simulink model "Ex2s"  (R2025a)
settings: Solver=VariableStepAuto  StartTime=0.0  StopTime=4  RelTol=1e-3

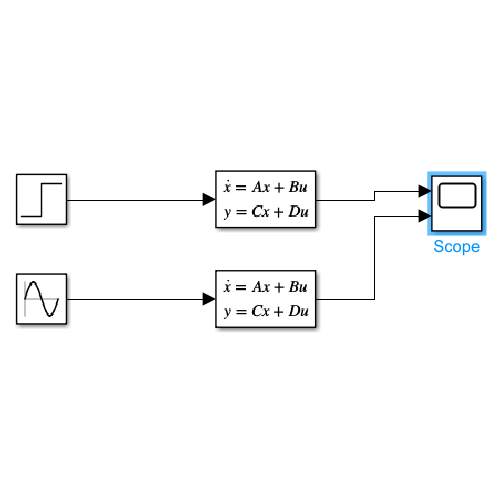
[thumbnail: Simulink's stored preview of the top-level diagram]
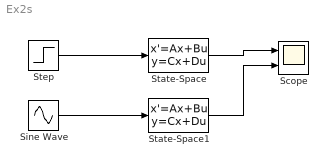
== system Ex2s ==
  Scope : Scope  NumInputPorts=2
      settings: ActiveDisplayYMinimum=-0.67263094426115744  ActiveDisplayYMaximum=2.2878733925560457
  Sine Wave : Sin  Frequency=2*pi  SampleTime=0
  State-Space : StateSpace  A=[0 1 0; 0 0 1; -6 -11 -6]  B=[1;1;1]  C=[1 1 0]  D=0  InitialCondition=[1; 0.5; -0.5]
  State-Space1 : StateSpace  A=[0 1 0; 0 0 1; -6 -11 -6]  B=[1;1;1]  C=[1 1 0]  D=0  InitialCondition=[1; 0.5; -0.5]
  Step : Step  SampleTime=0
  wires:
  Step/1 -> State-Space/1
  State-Space/1 -> Scope/1
  Sine Wave/1 -> State-Space1/1
  State-Space1/1 -> Scope/2
